simulink model "MATLAb_Func"  (R2012b)
settings: Solver=ode45  StartTime=0.0  StopTime=10  RelTol=1e-6
settings Model: Creator=Faradars  LastModifiedBy=Faradars

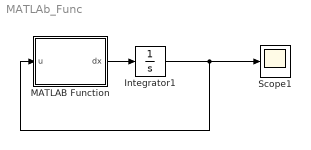
== system MATLAb_Func ==
  Integrator1 : Integrator  InitialCondition=[0.7;0;0]
  MATLAB Function : MATLAB Function  TreatAsAtomicUnit=on
  Scope1 : Scope
      settings: SaveName=chua1
  wires:
  Integrator1/1 -> MATLAB Function/1(u), Scope1/1
  MATLAB Function/1(dx) -> Integrator1/1

== matlab function MATLAb_Func/MATLAB Function ==
  data: u input; dx output
function dx = fcn(u)
%#codegen
x=u(1);
y=u(2);
z=u(3);

alpha=15.6;
beta=28;
m0=-1.143;
m1=-0.714;

h=m1*x+0.5*(m0-m1)*(abs(x+1)-abs(x-1));
xdot=alpha*(y-x-h);
ydot=x-y+z;
zdot=-beta*y;

dx=[xdot ydot zdot]';

end
